simulink model "updated_regelung"  (R2014a)
settings: Solver=ode45  StartTime=0.0  StopTime=10.0  RelTol=1e-3
undefined symbols (not defined in the file): c_we, F_g, F_l, h_l, h_r, J, m, schub_const, x_soll, y_soll, z_soll
settings Model: Creator=loren_000  LastModifiedBy=Administrator

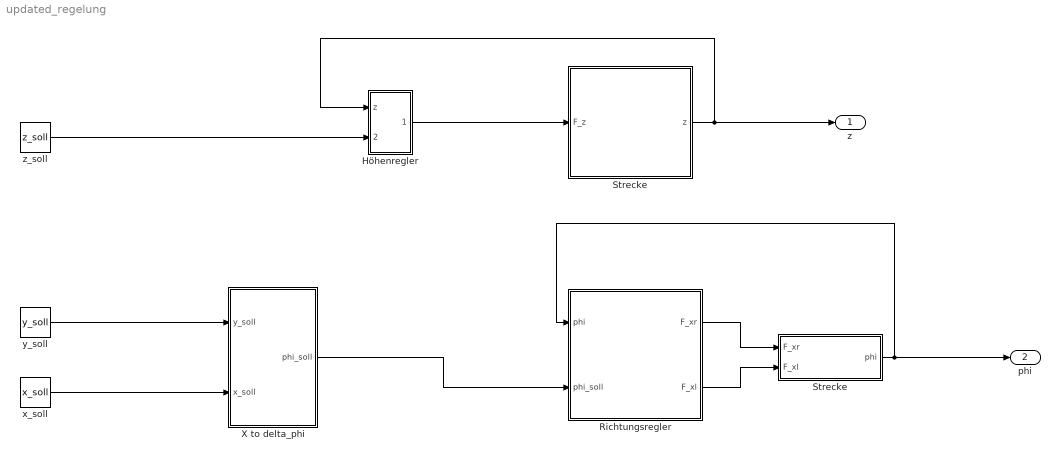
== system updated_regelung ==
  Höhenregler : Subsystem
  Richtungsregler : Subsystem
  Strecke : Subsystem
  "Strecke " : Subsystem
  X to delta_phi : Subsystem
  x_soll : Constant  Value=x_soll
  y_soll : Constant  Value=y_soll
  z_soll : Constant  Value=z_soll
  z : Outport
  phi : Outport  Port=2
  wires:
  z_soll/1 -> Höhenregler/2(z_soll)
  X to delta_phi/1(phi_soll) -> Richtungsregler/2(phi_soll)
  y_soll/1 -> X to delta_phi/1(y_soll)
  x_soll/1 -> X to delta_phi/2(x_soll)
  Höhenregler/1(F_z) -> "Strecke "/1(F_z)
  "Strecke "/1(z) -> z/1, Höhenregler/1(z)
  Richtungsregler/1(F_xr) -> Strecke/1(F_xr)
  Richtungsregler/2(F_xl) -> Strecke/2(F_xl)
  Strecke/1(phi) -> phi/1, Richtungsregler/1(phi)

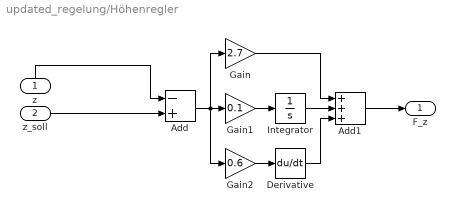
== system updated_regelung/Höhenregler ==
  z : Inport
  z_soll : Inport  Port=2
  Add : Sum  Inputs=-+
  Add1 : Sum  Inputs=+++
  Derivative : Derivative
  Gain : Gain  Gain=2.7
  Gain1 : Gain  Gain=0.1
  Gain2 : Gain  Gain=0.6
  Integrator : Integrator
  F_z : Outport
  wires:
  z/1 -> Add/1
  Integrator/1 -> Add1/2
  Derivative/1 -> Add1/3
  z_soll/1 -> Add/2
  Add/1 -> Gain2/1, Gain1/1, Gain/1
  Gain/1 -> Add1/1
  Add1/1 -> F_z/1
  Gain1/1 -> Integrator/1
  Gain2/1 -> Derivative/1

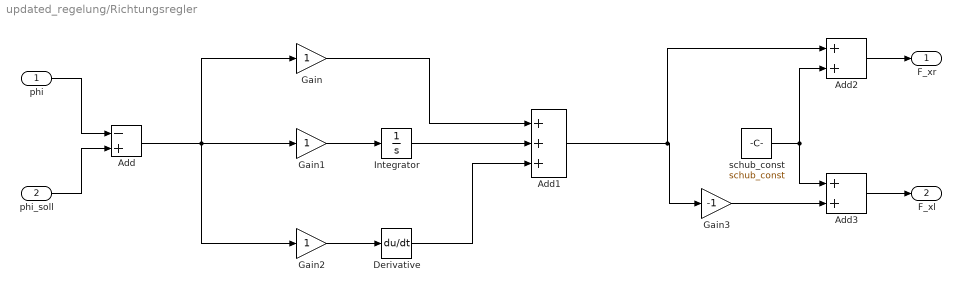
== system updated_regelung/Richtungsregler ==
  phi : Inport
  phi_soll : Inport  Port=2
  Add : Sum  Inputs=-+
  Add1 : Sum  Inputs=+++
  Add2 : Sum
  Add3 : Sum
  Derivative : Derivative
  Gain : Gain
  Gain1 : Gain
  Gain2 : Gain
  Gain3 : Gain  Gain=-1
  Integrator : Integrator
  schub_const : Constant  Value=schub_const
  F_xr : Outport
  F_xl : Outport  Port=2
  wires:
  phi/1 -> Add/1
  phi_soll/1 -> Add/2
  Add/1 -> Gain2/1, Gain/1, Gain1/1
  Gain1/1 -> Integrator/1
  Gain2/1 -> Derivative/1
  Gain/1 -> Add1/1
  Integrator/1 -> Add1/2
  Derivative/1 -> Add1/3
  Add1/1 -> Add2/1, Gain3/1
  Add2/1 -> F_xr/1
  schub_const/1 -> Add3/1, Add2/2
  Add3/1 -> F_xl/1
  Gain3/1 -> Add3/2

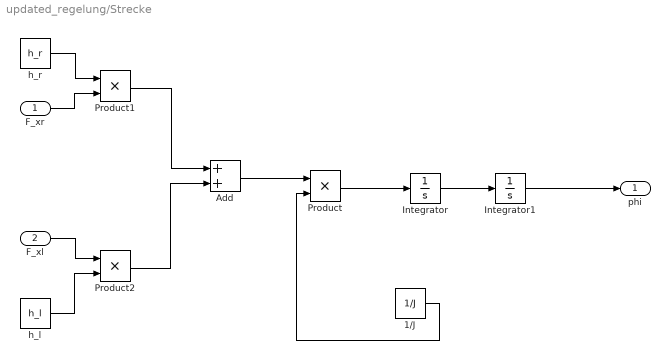
== system updated_regelung/Strecke ==
  F_xr : Inport
  F_xl : Inport  Port=2
  1/J : Constant  Value=1/J
  Add : Sum
  Integrator : Integrator
  Integrator1 : Integrator
  Product : Product
  Product1 : Product
  Product2 : Product
  h_l : Constant  Value=h_l
  h_r : Constant  Value=h_r
  phi : Outport
  wires:
  Integrator1/1 -> phi/1
  Integrator/1 -> Integrator1/1
  1/J/1 -> Product/2
  Add/1 -> Product/1
  Product/1 -> Integrator/1
  F_xl/1 -> Product2/1
  h_l/1 -> Product2/2
  F_xr/1 -> Product1/2
  h_r/1 -> Product1/1
  Product1/1 -> Add/1
  Product2/1 -> Add/2

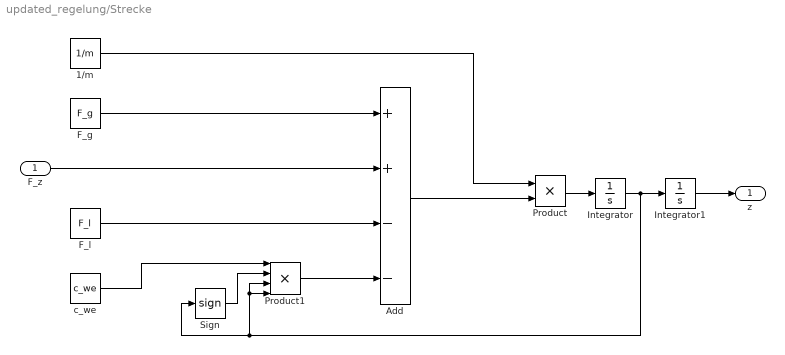
== system updated_regelung/Strecke  ==
  F_z : Inport
  1/m : Constant  Value=1/m
  Add : Sum  Inputs=++--
  F_g : Constant  Value=F_g
  F_l : Constant  Value=F_l
  Integrator : Integrator
  Integrator1 : Integrator
  Product : Product
  Product1 : Product  Inputs=4
  Sign : Signum
  c_we : Constant  Value=c_we
  z : Outport
  wires:
  Add/1 -> Product/2
  F_z/1 -> Add/2
  F_g/1 -> Add/1
  c_we/1 -> Product1/1
  Sign/1 -> Product1/2
  Integrator1/1 -> z/1
  Product/1 -> Integrator/1
  Integrator/1 -> Product1/3, Product1/4, Sign/1, Integrator1/1
  F_l/1 -> Add/3
  Product1/1 -> Add/4
  1/m/1 -> Product/1

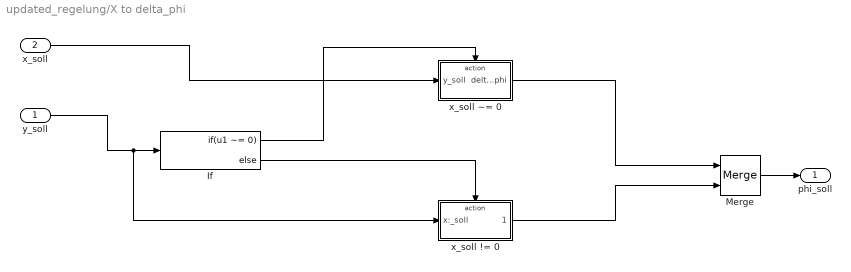
== system updated_regelung/X to delta_phi ==
  y_soll : Inport
  x_soll : Inport  Port=2
  If : If  IfExpression=u1 ~= 0
  Merge : Merge
  x_soll != 0 : Subsystem  TreatAsAtomicUnit=on
  x_soll ~= 0 : Subsystem  TreatAsAtomicUnit=on
  phi_soll : Outport
  wires:
  x_soll/1 -> x_soll ~= 0/1(y_soll)
  x_soll ~= 0/1(delta_phi) -> Merge/1
  x_soll != 0/1(delta_phi) -> Merge/2
  Merge/1 -> phi_soll/1
  If/1 -> x_soll ~= 0/Action
  If/2 -> x_soll != 0/Action
  y_soll/1 -> x_soll != 0/1(x:_soll), If/1

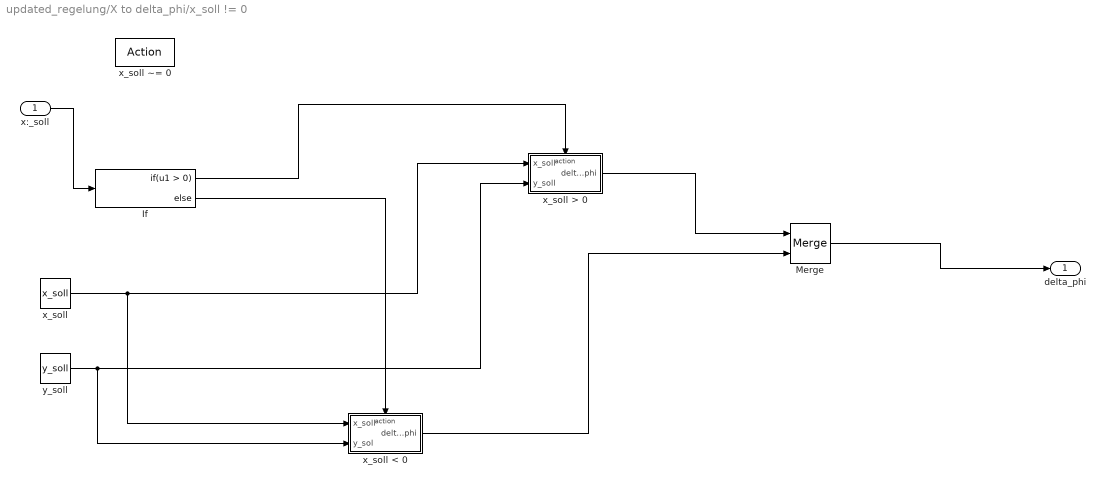
== system updated_regelung/X to delta_phi/x_soll != 0 ==
  x:_soll : Inport
  x_soll ~= 0 : ActionPort  ActionType=else
  If : If
  Merge : Merge
  "x_soll " : Constant  Value=x_soll
  x_soll < 0 : Subsystem  TreatAsAtomicUnit=on
  x_soll > 0 : Subsystem  TreatAsAtomicUnit=on
  y_soll : Constant  Value=y_soll
  delta_phi : Outport
  wires:
  x:_soll/1 -> If/1
  If/1 -> x_soll > 0/Action
  If/2 -> x_soll < 0/Action
  "x_soll "/1 -> x_soll < 0/1(x_soll), x_soll > 0/1("x_soll ")
  y_soll/1 -> x_soll < 0/2(y_sol), x_soll > 0/2(y_soll)
  x_soll > 0/1(delta_phi) -> Merge/1
  x_soll < 0/1(delta_phi) -> Merge/2
  Merge/1 -> delta_phi/1

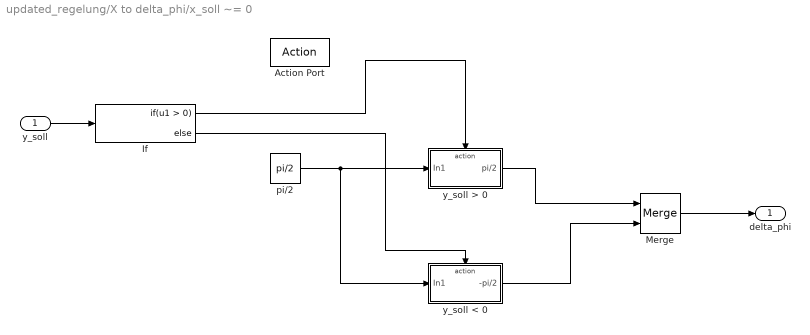
== system updated_regelung/X to delta_phi/x_soll ~= 0 ==
  y_soll : Inport
  Action Port : ActionPort  ActionType=then
  If : If
  Merge : Merge
  pi/2 : Constant  Value=pi/2
  y_soll < 0 : Subsystem  TreatAsAtomicUnit=on
  y_soll > 0 : Subsystem  TreatAsAtomicUnit=on
  delta_phi : Outport
  wires:
  y_soll/1 -> If/1
  If/1 -> y_soll > 0/Action
  pi/2/1 -> y_soll < 0/1(In1), y_soll > 0/1(In1)
  If/2 -> y_soll < 0/Action
  y_soll < 0/1(-pi/2) -> Merge/2
  y_soll > 0/1(pi/2) -> Merge/1
  Merge/1 -> delta_phi/1

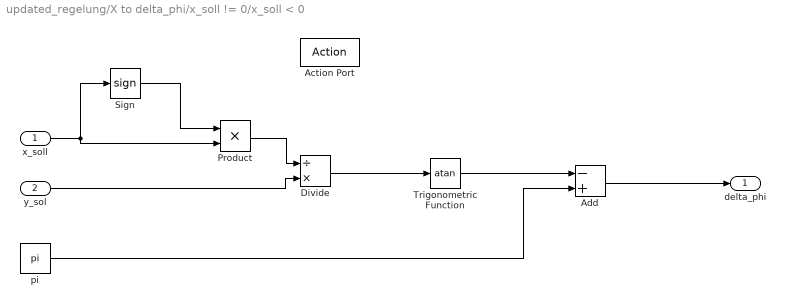
== system updated_regelung/X to delta_phi/x_soll != 0/x_soll < 0 ==
  x_soll : Inport
  y_sol : Inport  Port=2
  Action Port : ActionPort  ActionType=else
  Add : Sum  Inputs=-+
  Divide : Product  Inputs=/*
  Product : Product  Inputs=**
  Sign : Signum
  Trigonometric Function : Trigonometry  Operator=atan
  pi : Constant  Value=pi
  delta_phi : Outport
  wires:
  x_soll/1 -> Product/2, Sign/1
  Sign/1 -> Product/1
  Product/1 -> Divide/1
  y_sol/1 -> Divide/2
  Divide/1 -> Trigonometric Function/1
  Trigonometric Function/1 -> Add/1
  pi/1 -> Add/2
  Add/1 -> delta_phi/1

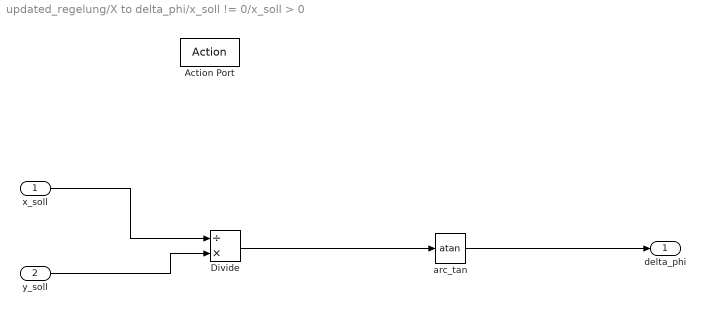
== system updated_regelung/X to delta_phi/x_soll != 0/x_soll > 0 ==
  "x_soll " : Inport
  y_soll : Inport  Port=2
  Action Port : ActionPort  ActionType=then
  Divide : Product  Inputs=/*
  arc_tan : Trigonometry  Operator=atan
  delta_phi : Outport
  wires:
  "x_soll "/1 -> Divide/1
  y_soll/1 -> Divide/2
  Divide/1 -> arc_tan/1
  arc_tan/1 -> delta_phi/1

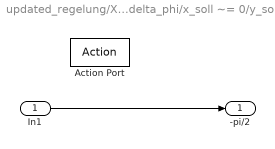
== system updated_regelung/X to delta_phi/x_soll ~= 0/y_soll < 0 ==
  In1 : Inport
  Action Port : ActionPort  ActionType=else
  -pi/2 : Outport
  wires:
  In1/1 -> -pi/2/1

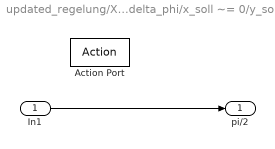
== system updated_regelung/X to delta_phi/x_soll ~= 0/y_soll > 0 ==
  In1 : Inport
  Action Port : ActionPort  ActionType=then
  pi/2 : Outport
  wires:
  In1/1 -> pi/2/1
